simulink model "EEG_2022_040_Simulink_ex4"  (R2024a)
settings: Solver=VariableStepAuto  StartTime=0.0  StopTime=10.0  RelTol=1e-3
model workspace (MAT data in the model file):
  wn = Simulink.Parameter
  wn.Complexity = 'real'
  wn.Dimensions = [0 0]
  wn.DataType = 'auto'
libraries: simulink x1
settings Model: Creator=User  LastModifiedBy=User

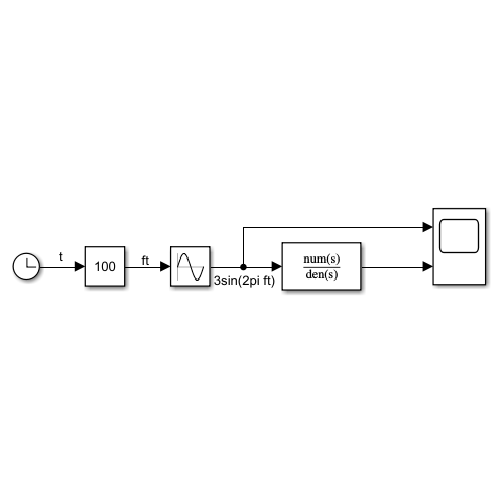
[thumbnail: Simulink's stored preview of the top-level diagram]
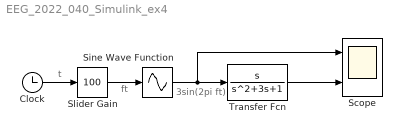
== system EEG_2022_040_Simulink_ex4 ==
  note: 3sin(2pi ft)
  note: ft
  note: t
  Clock : Clock
  Scope : Scope  NumInputPorts=2
  Sine Wave Function : Sin  TimeSource=Use external signal  SampleTime=0
  Slider Gain : simulink/Math Operations/Slider Gain  gain=100  low=0  high=100
  Transfer Fcn : TransferFcn  Numerator=[1 0]  Denominator=[1 3 1]  ParameterTunability=Unconstrained
  wires:
  Clock/1 -> Slider Gain/1
  Slider Gain/1 -> Sine Wave Function/1
  Sine Wave Function/1 -> Scope/1, Transfer Fcn/1
  Transfer Fcn/1 -> Scope/2
